simulink model "IMpanel"  (R2020a)
settings: Solver=ode45  StartTime=0.0  StopTime=10.0  FixedStep=5e-6  RelTol=1e-6  AbsTol=1e-8
values from neighbouring files (symbols this model uses):
  B = 0.08    [Mainprog.m]
  Ba = alphas * Jhat - Bhat    (= 0.17)    [Mainprog.m]
  Cdc = 5*470e-6    (= 0.00235)    [Mainprog.m]
  Flux_ref = 0.66*sqrt(2)*Lm/Lr    [Mainprog.m]
  Flux_ref_time = 0.001    [Mainprog.m]
  Israted = 9.1*sqrt(2)*1.2    [Mainprog.m]
  J = 0.05*0.25    (= 0.0125)    [Mainprog.m]
  kic = alphac * (RRhat + Rshat + Ra)    (= 15552.4475524)    [Mainprog.m]
  kis = alphas * (Bhat + Ba)    (= 5)    [Mainprog.m]
  kpc = alphac * Lsigmahat    (= 15.5524475524)    [Mainprog.m]
  kps = alphas * Jhat    (= 0.25)    [Mainprog.m]
  Lm = 0.135    [Mainprog.m]
  LMhat = LM    (= 0.127447552448)    [Mainprog.m]
  Lr = Lm+Lrl    (= 0.143)    [Mainprog.m]    (also in asymach.m = Lm+Lrl)
  Lrl = 0.008    [Mainprog.m]
  Lsigmahat = Lsigma    (= 0.0155524475524)    [Mainprog.m]
  Lsl = 0.008    [Mainprog.m]
  np = 2    [Mainprog.m]
  Ra = Lsigmahat * alphac - Rshat - RRhat    (= 13.1173079368)    [Mainprog.m]
  Rbatt = 1    [Mainprog.m]
  RR = (Lm/Lr)^2*Rr    (= 1.10513961563)    [Mainprog.m]
  Rr = 1.24    [Mainprog.m]
  RRhat = RR    (= 1.10513961563)    [Mainprog.m]
  Rs = 1.33    [Mainprog.m]
  speed_ref = 1435*pi/30    (= 150.272848597)    [Mainprog.m]
  speed_ref_time = 0.5    [Mainprog.m]
  Te_ref_time = 0.5    [Mainprog.m]
  Te_ref_value = 12    [Mainprog.m]
  TL_extra = 14.4    [Mainprog.m]    (also in asymach.m = u(3))
  TL_extra_time = 1    [Mainprog.m]
  Ts = 1/5000    (= 0.0002)    [Mainprog.m]
  Vbatt = 625    [Mainprog.m]
  Vdc0 = Vbatt    (= 625)    [Mainprog.m]
  xi = [0;0;0;0;0;0]    [Mainprog.m]
undefined symbols (not defined in the file or in its folder): j
libraries: simulink x1
settings Model: ExtModeTrigMode=oneshot  ExtModeArmWhenConnect=off  ExtModeAutoUpdateStatusClock=off  Creator=e6zebra  LastModifiedBy=miche
settings SolverCC: AutoScaleAbsTol=off
settings DataIOCC: SaveFormat=Array  SignalLoggingSaveFormat=ModelDataLogs  ReturnWorkspaceOutputs=off
settings OptimizationCC: BlockReduction=off  BooleanDataType=off  ExpressionDepthLimit=2147483647  InitFltsAndDblsToZero=on  LifeSpan=inf
settings DebuggingCC: SaveWithParameterizedLinksMsg=none  UnderspecifiedInitializationDetection=Classic  MergeDetectMultiDrivingBlocksExec=none  SignalResolutionControl=TryResolveAllWithWarning  MultiTaskDSMMsg=warning  MultiTaskCondExecSysMsg=none  FcnCallInpInsideContextMsg=warning  StateNameClashWarn=warning  SFUnexpectedBacktrackingDiag=warning  SFNoUnconditionalDefaultTransitionDiag=warning  SFExecutionAtInitializationDiag=none  ArithmeticOperatorsInVariantConditions=warning
settings HardwareCC: ProdBitPerPointer=32  ProdBitPerSizeT=32  ProdBitPerPtrDiffT=32  ProdLargestAtomicFloat=None  ProdIntDivRoundTo=Undefined  ProdEndianess=Unspecified  ProdWordSize=32  ProdHWDeviceType=32-bit Generic  TargetUnknown=on
settings ModelReferenceCC: PropagateSignalLabelsOutOfModel=off
settings SFSimCC: SimUseLocalCustomCode=off  CustomCodeUndefinedFunction=UseInterfaceOnly
settings RTWCC: TemplateMakefile=grt.tmf  RTWUseLocalCustomCode=off
settings CodeAppCC: StateflowObjectComments=on
settings GRTTargetCC: TargetFcnLib=ansi_tfl_tmw.mat  TargetLangStandard=C89/C90 (ANSI)  CombineOutputUpdateFcns=off  GRTInterface=on
settings ConfigComp: CovMetricSettings=dw  CovHtmlReporting=on  CovSaveCumulativeToWorkspaceVar=on  CovSaveSingleToWorkspaceVar=on  CovExternalEMLEnable=off  CovSFcnEnable=off

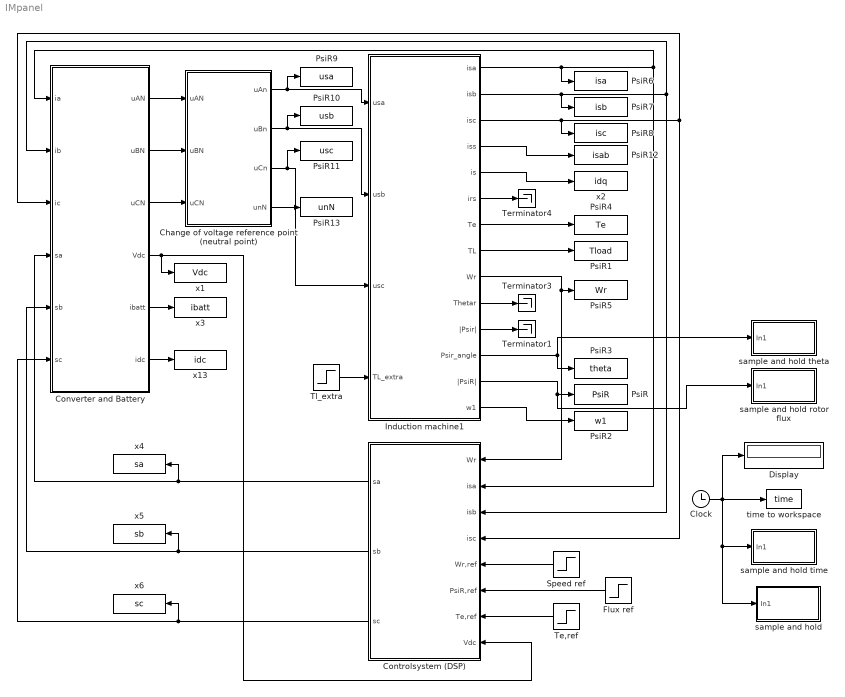
== system IMpanel ==
  Change of voltage reference point (neutral point) : Subsystem
  Clock : Clock
  Controlsystem (DSP) : Subsystem  TreatAsAtomicUnit=on
  Converter and Battery : Subsystem
  Display : Display
  Flux ref : Step  Time=Flux_ref_time  After=Flux_ref  SampleTime=0
  Induction machine1 : Subsystem
  PsiR : ToWorkspace  VariableName=PsiR  SampleTime=-1
  PsiR1 : ToWorkspace  VariableName=Tload  SampleTime=-1
  PsiR10 : ToWorkspace  VariableName=usb  SampleTime=-1
  PsiR11 : ToWorkspace  VariableName=usc  SampleTime=-1
  PsiR12 : ToWorkspace  VariableName=isab  SampleTime=-1
  PsiR13 : ToWorkspace  VariableName=unN  SampleTime=-1
  PsiR2 : ToWorkspace  VariableName=w1  SampleTime=-1
  PsiR3 : ToWorkspace  VariableName=theta  SampleTime=-1
  PsiR4 : ToWorkspace  VariableName=Te  SampleTime=-1
  PsiR5 : ToWorkspace  VariableName=Wr  SampleTime=-1
  PsiR6 : ToWorkspace  VariableName=isa  SampleTime=-1
  PsiR7 : ToWorkspace  VariableName=isb  SampleTime=-1
  PsiR8 : ToWorkspace  VariableName=isc  SampleTime=-1
  PsiR9 : ToWorkspace  VariableName=usa  SampleTime=-1
  Speed ref : Step  Time=speed_ref_time  After=speed_ref  SampleTime=0
  Te,ref : Step  Time=Te_ref_time  After=Te_ref_value  SampleTime=0
  Terminator1 : Terminator
  Terminator3 : Terminator
  Terminator4 : Terminator
  Tl_extra : Step  Time=TL_extra_time  After=TL_extra  SampleTime=0
  sample and hold : Subsystem
  sample and hold rotor flux : Subsystem
  sample and hold theta : Subsystem
  sample and hold time : Subsystem
  time to workspace : ToWorkspace  VariableName=time  SampleTime=-1
  x1 : ToWorkspace  VariableName=Vdc  SampleTime=-1
  x13 : ToWorkspace  VariableName=idc  SampleTime=-1
  x2 : ToWorkspace  VariableName=idq  SampleTime=-1
  x3 : ToWorkspace  VariableName=ibatt  SampleTime=-1
  x4 : ToWorkspace  VariableName=sa  SampleTime=-1
  x5 : ToWorkspace  VariableName=sb  SampleTime=-1
  x6 : ToWorkspace  VariableName=sc  SampleTime=-1
  wires:
  Clock/1 -> time to workspace/1, Display/1, sample and hold/1(In1), sample and hold time/1(In1)
  Induction machine1/13(|PsiR|) -> sample and hold rotor flux/1(In1), PsiR/1
  Induction machine1/9(Wr) -> Controlsystem (DSP)/1(Wr), PsiR5/1
  Induction machine1/3(isc) -> PsiR8/1, Controlsystem (DSP)/4(isc), Converter and Battery/3(ic)
  Induction machine1/2(isb) -> PsiR7/1, Controlsystem (DSP)/3(isb), Converter and Battery/2(ib)
  Induction machine1/1(isa) -> PsiR6/1, Controlsystem (DSP)/2(isa), Converter and Battery/1(ia)
  Flux ref/1 -> Controlsystem (DSP)/6(PsiR,ref)
  Speed ref/1 -> Controlsystem (DSP)/5(Wr,ref)
  Te,ref/1 -> Controlsystem (DSP)/7(Te,ref)
  Converter and Battery/5(ibatt) -> x3/1
  Converter and Battery/6(idc) -> x13/1
  Converter and Battery/4(Vdc) -> Controlsystem (DSP)/8(Vdc), x1/1
  Controlsystem (DSP)/1(sa) -> x4/1, Converter and Battery/4(sa)
  Controlsystem (DSP)/2(sb) -> x5/1, Converter and Battery/5(sb)
  Controlsystem (DSP)/3(sc) -> x6/1, Converter and Battery/6(sc)
  Converter and Battery/1(uAN) -> Change of voltage reference point (neutral point)/1(uAN)
  Converter and Battery/2(uBN) -> Change of voltage reference point (neutral point)/2(uBN)
  Converter and Battery/3(uCN) -> Change of voltage reference point (neutral point)/3(uCN)
  Change of voltage reference point (neutral point)/1(uAn) -> PsiR9/1, Induction machine1/1(usa)
  Change of voltage reference point (neutral point)/2(uBn) -> PsiR10/1, Induction machine1/2(usb)
  Change of voltage reference point (neutral point)/3(uCn) -> PsiR11/1, Induction machine1/3(usc)
  Change of voltage reference point (neutral point)/4(unN) -> PsiR13/1
  Induction machine1/7(Te) -> PsiR4/1
  Tl_extra/1 -> Induction machine1/4(TL_extra)
  Induction machine1/4(iss) -> PsiR12/1
  Induction machine1/5(is) -> x2/1
  Induction machine1/14(w1) -> PsiR2/1
  Induction machine1/8(TL) -> PsiR1/1
  Induction machine1/12(Psir_angle) -> sample and hold theta/1(In1), PsiR3/1
  Induction machine1/11(|Psir|) -> Terminator1/1
  Induction machine1/10(Thetar) -> Terminator3/1
  Induction machine1/6(irs) -> Terminator4/1

== system IMpanel/Change of voltage reference point (neutral point) ==
  uAN : Inport
  uBN : Inport  Port=2
  uCN : Inport  Port=3
  Gain2 : Gain  Gain=1/3  SaturateOnIntegerOverflow=on  OutDataTypeStr=Inherit: Same as input  ParamDataTypeStr=Inherit: Same as input
  Sum1 : Sum  Inputs=|+-  SaturateOnIntegerOverflow=on
  Sum4 : Sum  Inputs=|+-  SaturateOnIntegerOverflow=on
  Sum5 : Sum  Inputs=|+-  SaturateOnIntegerOverflow=on
  Sum7 : Sum  Inputs=+++  SaturateOnIntegerOverflow=on
  uAn : Outport  VectorParamsAs1DForOutWhenUnconnected=off
  uBn : Outport  Port=2  VectorParamsAs1DForOutWhenUnconnected=off
  uCn : Outport  Port=3  VectorParamsAs1DForOutWhenUnconnected=off
  unN : Outport  Port=4  VectorParamsAs1DForOutWhenUnconnected=off
  wires:
  uCN/1 -> Sum5/1, Sum7/1
  uBN/1 -> Sum4/1, Sum7/2
  uAN/1 -> Sum1/1, Sum7/3
  Sum7/1 -> Gain2/1
  Gain2/1 -> Sum1/2, Sum4/2, Sum5/2, unN/1
  Sum1/1 -> uAn/1
  Sum4/1 -> uBn/1
  Sum5/1 -> uCn/1

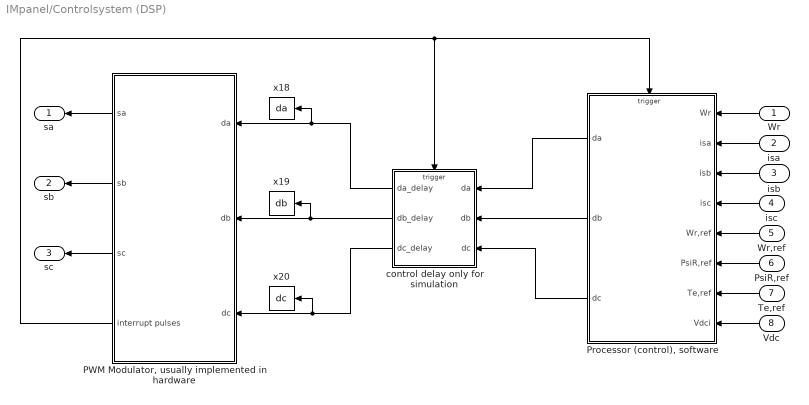
== system IMpanel/Controlsystem (DSP) ==
  Wr : Inport
  isa : Inport  Port=2
  isb : Inport  Port=3
  isc : Inport  Port=4
  Wr,ref : Inport  Port=5
  PsiR,ref : Inport  Port=6
  Te,ref : Inport  Port=7
  Vdc : Inport  Port=8
  "PWM Modulator, usually implemented in hardware" : Subsystem
  "Processor (control), software" : Subsystem  TreatAsAtomicUnit=on
  control delay only for simulation : Subsystem  TreatAsAtomicUnit=on
  x18 : ToWorkspace  VariableName=da  SampleTime=-1
  x19 : ToWorkspace  VariableName=db  SampleTime=-1
  x20 : ToWorkspace  VariableName=dc  SampleTime=-1
  sa : Outport  VectorParamsAs1DForOutWhenUnconnected=off
  sb : Outport  Port=2  VectorParamsAs1DForOutWhenUnconnected=off
  sc : Outport  Port=3  VectorParamsAs1DForOutWhenUnconnected=off
  wires:
  "PWM Modulator, usually implemented in hardware"/1(sa) -> sa/1
  "PWM Modulator, usually implemented in hardware"/2(sb) -> sb/1
  "PWM Modulator, usually implemented in hardware"/3(sc) -> sc/1
  Vdc/1 -> "Processor (control), software"/8(Vdci)
  Te,ref/1 -> "Processor (control), software"/7(Te,ref)
  PsiR,ref/1 -> "Processor (control), software"/6(PsiR,ref)
  Wr,ref/1 -> "Processor (control), software"/5(Wr,ref)
  Wr/1 -> "Processor (control), software"/1(Wr)
  isa/1 -> "Processor (control), software"/2(isa)
  isb/1 -> "Processor (control), software"/3(isb)
  isc/1 -> "Processor (control), software"/4(isc)
  "PWM Modulator, usually implemented in hardware"/4("interrupt pulses ") -> "Processor (control), software"/Trigger, control delay only for simulation/Trigger
  "Processor (control), software"/1(da) -> control delay only for simulation/1(da)
  control delay only for simulation/1(da_delay) -> x18/1, "PWM Modulator, usually implemented in hardware"/1(da)
  "Processor (control), software"/2(db) -> control delay only for simulation/2(db)
  control delay only for simulation/2(db_delay) -> x19/1, "PWM Modulator, usually implemented in hardware"/2(db)
  "Processor (control), software"/3(dc) -> control delay only for simulation/3(dc)
  control delay only for simulation/3(dc_delay) -> x20/1, "PWM Modulator, usually implemented in hardware"/3(dc)

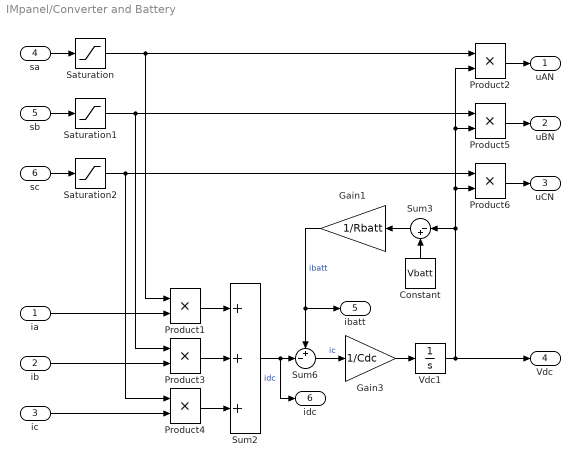
== system IMpanel/Converter and Battery ==
  ia : Inport
  ib : Inport  Port=2
  ic : Inport  Port=3
  sa : Inport  Port=4
  sb : Inport  Port=5
  sc : Inport  Port=6
  Constant : Constant  Value=Vbatt
  Gain1 : Gain  Gain=1/Rbatt  SaturateOnIntegerOverflow=on  OutDataTypeStr=Inherit: Same as input  ParamDataTypeStr=Inherit: Same as input
  Gain3 : Gain  Gain=1/Cdc  SaturateOnIntegerOverflow=on  OutDataTypeStr=Inherit: Same as input  ParamDataTypeStr=Inherit: Same as input
  Product{1..6} (6 alike) : Product  SaturateOnIntegerOverflow=on  OutDataTypeStr=Inherit: Same as first input
  Saturation : Saturate  UpperLimit=1.0  LowerLimit=0.0
  Saturation1 : Saturate  UpperLimit=1.0  LowerLimit=0.0
  Saturation2 : Saturate  UpperLimit=1.0  LowerLimit=0.0
  Sum2 : Sum  Inputs=+++  SaturateOnIntegerOverflow=on
  Sum3 : Sum  Inputs=|-+  SaturateOnIntegerOverflow=on
  Sum6 : Sum  Inputs=+-|  SaturateOnIntegerOverflow=on
  Vdc1 : Integrator  InitialCondition=Vdc0  LimitOutput=on  LowerSaturationLimit=1
  uAN : Outport  VectorParamsAs1DForOutWhenUnconnected=off
  uBN : Outport  Port=2  VectorParamsAs1DForOutWhenUnconnected=off
  uCN : Outport  Port=3  VectorParamsAs1DForOutWhenUnconnected=off
  Vdc : Outport  Port=4  VectorParamsAs1DForOutWhenUnconnected=off
  ibatt : Outport  Port=5  VectorParamsAs1DForOutWhenUnconnected=off
  idc : Outport  Port=6  VectorParamsAs1DForOutWhenUnconnected=off
  wires:
  Product2/1 -> uAN/1
  ic/1 -> Product4/2
  ib/1 -> Product3/2
  ia/1 -> Product1/2
  sa/1 -> Saturation/1
  sb/1 -> Saturation1/1
  sc/1 -> Saturation2/1
  Saturation2/1 -> Product4/1, Product6/1
  Saturation1/1 -> Product3/1, Product5/1
  Saturation/1 -> Product1/1, Product2/1
  Vdc1/1 -> Vdc/1, Sum3/1, Product6/2, Product5/2, Product2/2
  Constant/1 -> Sum3/2
  Product5/1 -> uBN/1
  Product6/1 -> uCN/1
  Product1/1 -> Sum2/1
  Product3/1 -> Sum2/2
  Product4/1 -> Sum2/3
  Sum3/1 -> Gain1/1
  Sum6/1 -> Gain3/1  "ic"
  Sum2/1 -> Sum6/2, idc/1  "idc"
  Gain1/1 -> Sum6/1, ibatt/1  "ibatt"
  Gain3/1 -> Vdc1/1

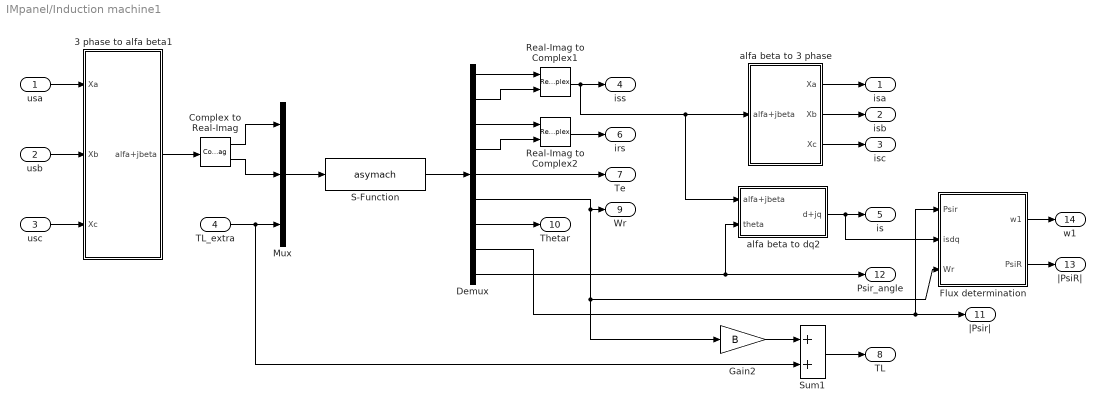
== system IMpanel/Induction machine1 ==
  usa : Inport
  usb : Inport  Port=2
  usc : Inport  Port=3
  TL_extra : Inport  Port=4
  3 phase to alfa beta1 : Subsystem
  Complex to Real-Imag : ComplexToRealImag
  Demux : Demux  Outputs=9
      settings: DisplayOption=none
  Flux determination : Subsystem
  Gain2 : Gain  Gain=B
  Mux : Mux  Inputs=3
  Real-Imag to Complex1 : RealImagToComplex
  Real-Imag to Complex2 : RealImagToComplex
  S-Function : S-Function  FunctionName=asymach  Parameters=Rs,Rr,Lm,Lsl,Lrl,J,np,B,xi  SFunctionDeploymentMode=off  EnableBusSupport=off
  Sum1 : Sum  InputSameDT=on  SaturateOnIntegerOverflow=on  OutDataTypeStr=Inherit: Same as first input
  alfa beta to 3 phase : Subsystem
  alfa beta to dq2 : Subsystem
  isa : Outport  VectorParamsAs1DForOutWhenUnconnected=off
  isb : Outport  Port=2  VectorParamsAs1DForOutWhenUnconnected=off
  isc : Outport  Port=3  VectorParamsAs1DForOutWhenUnconnected=off
  iss : Outport  Port=4  VectorParamsAs1DForOutWhenUnconnected=off
  is : Outport  Port=5  VectorParamsAs1DForOutWhenUnconnected=off
  irs : Outport  Port=6  VectorParamsAs1DForOutWhenUnconnected=off
  Te : Outport  Port=7  VectorParamsAs1DForOutWhenUnconnected=off
  TL : Outport  Port=8  VectorParamsAs1DForOutWhenUnconnected=off
  Wr : Outport  Port=9  VectorParamsAs1DForOutWhenUnconnected=off
  Thetar : Outport  Port=10  VectorParamsAs1DForOutWhenUnconnected=off
  |Psir| : Outport  Port=11  VectorParamsAs1DForOutWhenUnconnected=off
  Psir_angle : Outport  Port=12  VectorParamsAs1DForOutWhenUnconnected=off
  |PsiR| : Outport  Port=13  VectorParamsAs1DForOutWhenUnconnected=off
  w1 : Outport  Port=14  VectorParamsAs1DForOutWhenUnconnected=off
  wires:
  TL_extra/1 -> Mux/3, Sum1/2
  S-Function/1 -> Demux/1
  Mux/1 -> S-Function/1
  Demux/1 -> Real-Imag to Complex1/1
  Demux/2 -> Real-Imag to Complex1/2
  Real-Imag to Complex1/1 -> iss/1, alfa beta to dq2/1(alfa+jbeta), alfa beta to 3 phase/1(alfa+jbeta)
  Demux/3 -> Real-Imag to Complex2/1
  Demux/4 -> Real-Imag to Complex2/2
  Complex to Real-Imag/2 -> Mux/2
  Complex to Real-Imag/1 -> Mux/1
  alfa beta to dq2/1(d+jq) -> is/1, Flux determination/2(isdq)
  Real-Imag to Complex2/1 -> irs/1
  Demux/5 -> Te/1
  Sum1/1 -> TL/1
  Gain2/1 -> Sum1/1
  Demux/6 -> Wr/1, Gain2/1, Flux determination/3(Wr)
  Demux/7 -> Thetar/1
  Demux/9 -> alfa beta to dq2/2(theta), Psir_angle/1
  Demux/8 -> |Psir|/1, Flux determination/1(Psir)
  3 phase to alfa beta1/1(alfa+jbeta) -> Complex to Real-Imag/1
  usc/1 -> 3 phase to alfa beta1/3(Xc)
  usb/1 -> 3 phase to alfa beta1/2(Xb)
  usa/1 -> 3 phase to alfa beta1/1(Xa)
  alfa beta to 3 phase/1(Xa) -> isa/1
  alfa beta to 3 phase/3(Xc) -> isc/1
  alfa beta to 3 phase/2(Xb) -> isb/1
  Flux determination/2(PsiR) -> |PsiR|/1
  Flux determination/1(w1) -> w1/1

== system IMpanel/sample and hold ==
  In1 : Inport
  Pulse Generator : DiscretePulseGenerator  PulseType=Time based  Period=Ts/2  PulseWidth=50
  control : Subsystem  TreatAsAtomicUnit=on
  wires:
  Pulse Generator/1 -> control/Trigger
  In1/1 -> control/1(in)

== system IMpanel/sample and hold rotor flux ==
  In1 : Inport
  Pulse Generator : DiscretePulseGenerator  PulseType=Time based  Period=Ts  PulseWidth=50
  control : Subsystem  TreatAsAtomicUnit=on
  wires:
  In1/1 -> control/1(in)
  Pulse Generator/1 -> control/Trigger

== system IMpanel/sample and hold theta ==
  In1 : Inport
  Pulse Generator : DiscretePulseGenerator  PulseType=Time based  Period=Ts  PulseWidth=50
  control : Subsystem  TreatAsAtomicUnit=on
  wires:
  Pulse Generator/1 -> control/Trigger
  In1/1 -> control/1(in)

== system IMpanel/sample and hold time ==
  In1 : Inport
  Pulse Generator : DiscretePulseGenerator  PulseType=Time based  Period=Ts  PulseWidth=50
  control : Subsystem  TreatAsAtomicUnit=on
  wires:
  Pulse Generator/1 -> control/Trigger
  In1/1 -> control/1(in)

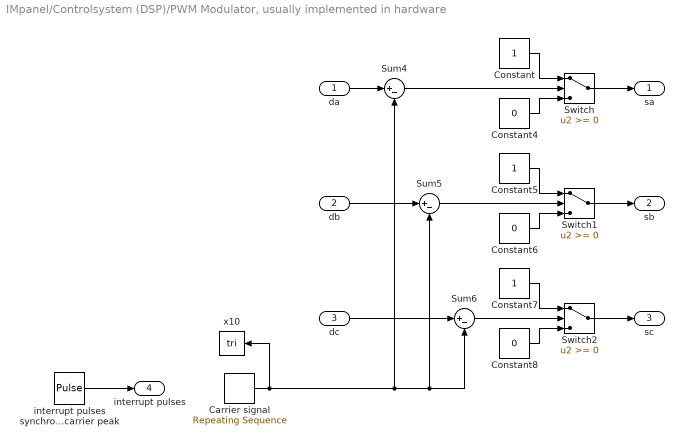
== system IMpanel/Controlsystem (DSP)/PWM Modulator, usually implemented in hardware ==
  da : Inport
  db : Inport  Port=2
  dc : Inport  Port=3
  Carrier signal : simulink/Sources/Repeating Sequence  rep_seq_t=[0 Ts/2 Ts]  rep_seq_y=[0 1 0]
  Constant : Constant
  Constant4 : Constant  Value=0
  Constant5 : Constant
  Constant6 : Constant  Value=0
  Constant7 : Constant
  Constant8 : Constant  Value=0
  Sum4 : Sum  Inputs=|+-
  Sum5 : Sum  Inputs=|+-
  Sum6 : Sum  Inputs=|+-
  Switch : Switch
  Switch1 : Switch
  Switch2 : Switch
  interrupt pulses synchronized with the carrier peak : DiscretePulseGenerator  PulseType=Time based  Period=Ts  PulseWidth=50
  x10 : ToWorkspace  VariableName=tri  SampleTime=-1
  sa : Outport  VectorParamsAs1DForOutWhenUnconnected=off
  sb : Outport  Port=2  VectorParamsAs1DForOutWhenUnconnected=off
  sc : Outport  Port=3  VectorParamsAs1DForOutWhenUnconnected=off
  "interrupt pulses " : Outport  Port=4  VectorParamsAs1DForOutWhenUnconnected=off
  wires:
  Constant/1 -> Switch/1
  Constant4/1 -> Switch/3
  Sum4/1 -> Switch/2
  Constant5/1 -> Switch1/1
  Constant6/1 -> Switch1/3
  Sum5/1 -> Switch1/2
  Constant7/1 -> Switch2/1
  Constant8/1 -> Switch2/3
  Sum6/1 -> Switch2/2
  Carrier signal/1 -> Sum6/2, Sum5/2, Sum4/2, x10/1
  Switch/1 -> sa/1
  Switch2/1 -> sc/1
  Switch1/1 -> sb/1
  da/1 -> Sum4/1
  db/1 -> Sum5/1
  dc/1 -> Sum6/1
  interrupt pulses synchronized with the carrier peak/1 -> "interrupt pulses "/1

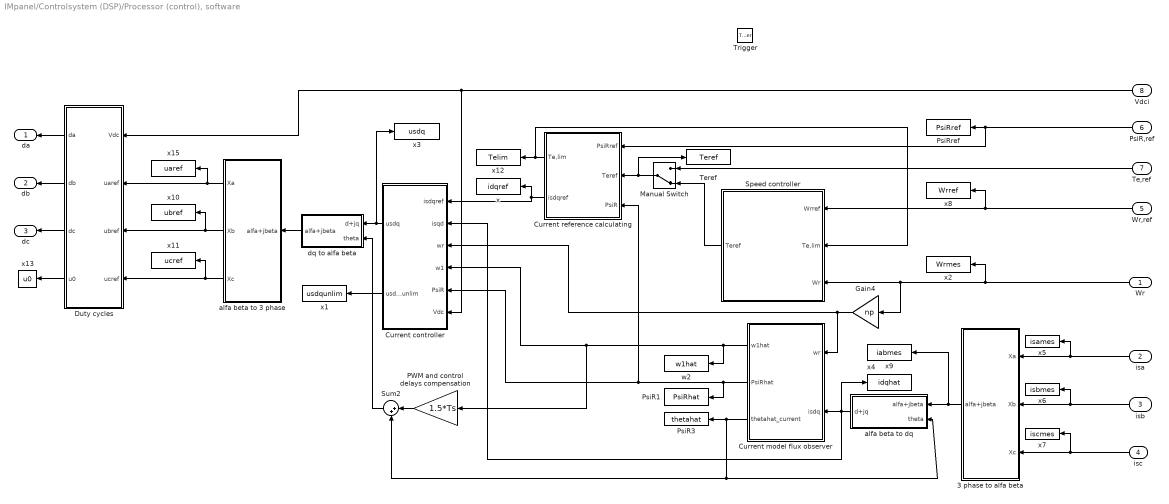
== system IMpanel/Controlsystem (DSP)/Processor (control), software ==
  Wr : Inport
  isa : Inport  Port=2
  isb : Inport  Port=3
  isc : Inport  Port=4
  Wr,ref : Inport  Port=5
  PsiR,ref : Inport  Port=6
  Te,ref : Inport  Port=7
  Vdci : Inport  Port=8
  Trigger : TriggerPort  VariantControl=(inherit)
  " Current model flux observer" : Subsystem
  3 phase to alfa beta : Subsystem
  Current controller : Subsystem
  Current reference calculating : Subsystem
  Duty cycles : Subsystem
  Gain4 : Gain  Gain=np  SaturateOnIntegerOverflow=on  OutDataTypeStr=Inherit: Same as input  ParamDataTypeStr=Inherit: Same as input
  Manual Switch : ManualSwitch  CurrentSetting=0
  PWM and control delays compensation : Gain  Gain=1.5*Ts  SaturateOnIntegerOverflow=on  OutDataTypeStr=Inherit: Same as input  ParamDataTypeStr=Inherit: Same as input
  PsiR1 : ToWorkspace  VariableName=PsiRhat  SampleTime=-1
  PsiR3 : ToWorkspace  VariableName=thetahat  SampleTime=-1
  PsiRref : ToWorkspace  VariableName=PsiRref  SampleTime=-1
  Speed controller : Subsystem
  Sum2 : Sum  Inputs=|++  SaturateOnIntegerOverflow=on
  Teref : ToWorkspace  VariableName=Teref  SampleTime=-1
  alfa beta to 3 phase : Subsystem
  alfa beta to dq : Subsystem
  dq to alfa beta : Subsystem
  w2 : ToWorkspace  VariableName=w1hat  SampleTime=-1
  x : ToWorkspace  VariableName=idqref  SampleTime=-1
  x1 : ToWorkspace  VariableName=usdqunlim  SampleTime=-1
  x10 : ToWorkspace  VariableName=ubref  SampleTime=-1
  x11 : ToWorkspace  VariableName=ucref  SampleTime=-1
  x12 : ToWorkspace  VariableName=Telim  SampleTime=-1
  x13 : ToWorkspace  VariableName=u0  SampleTime=-1
  x15 : ToWorkspace  VariableName=uaref  SampleTime=-1
  x2 : ToWorkspace  VariableName=Wrmes  SampleTime=-1
  x3 : ToWorkspace  VariableName=usdq  SampleTime=-1
  x4 : ToWorkspace  VariableName=idqhat  SampleTime=-1
  x5 : ToWorkspace  VariableName=isames  SampleTime=-1
  x6 : ToWorkspace  VariableName=isbmes  SampleTime=-1
  x7 : ToWorkspace  VariableName=iscmes  SampleTime=-1
  x8 : ToWorkspace  VariableName=Wrref  SampleTime=-1
  x9 : ToWorkspace  VariableName=iabmes  SampleTime=-1
  da : Outport  VectorParamsAs1DForOutWhenUnconnected=off
  db : Outport  Port=2  VectorParamsAs1DForOutWhenUnconnected=off
  dc : Outport  Port=3  VectorParamsAs1DForOutWhenUnconnected=off
  wires:
  Current controller/1(usdq) -> x3/1, dq to alfa beta/1(d+jq)
  " Current model flux observer"/2(PsiRhat) -> Current controller/5(PsiR), Current reference calculating/3(PsiR), PsiR1/1
  " Current model flux observer"/1(w1hat) -> w2/1, Current controller/4(w1), PWM and control delays compensation/1
  dq to alfa beta/1(alfa+jbeta) -> alfa beta to 3 phase/1(alfa+jbeta)
  Current controller/2(usdq unlim) -> x1/1
  alfa beta to dq/1(d+jq) -> " Current model flux observer"/2(isdq), x4/1, Current controller/2(isqd)
  Current reference calculating/1(Te,lim) -> Speed controller/2(Te,lim), x12/1
  Wr,ref/1 -> Speed controller/1(Wrref), x8/1
  3 phase to alfa beta/1(alfa+jbeta) -> alfa beta to dq/1(alfa+jbeta), x9/1
  Wr/1 -> x2/1, Speed controller/3(Wr), Gain4/1
  " Current model flux observer"/3(thetahat_current) -> PsiR3/1, Sum2/2, alfa beta to dq/2(theta)
  alfa beta to 3 phase/3(Xc) -> x11/1, Duty cycles/4(ucref)
  alfa beta to 3 phase/2(Xb) -> Duty cycles/3(ubref), x10/1
  alfa beta to 3 phase/1(Xa) -> x15/1, Duty cycles/2(uaref)
  Vdci/1 -> Duty cycles/1(Vdc), Current controller/6(Vdc)
  Gain4/1 -> Current controller/3(wr), " Current model flux observer"/1(wr)
  Manual Switch/1 -> Current reference calculating/2(Teref), Teref/1
  Speed controller/1(Teref) -> Manual Switch/2
  Te,ref/1 -> Manual Switch/1
  isa/1 -> 3 phase to alfa beta/1(Xa), x5/1
  isb/1 -> 3 phase to alfa beta/2(Xb), x6/1
  isc/1 -> 3 phase to alfa beta/3(Xc), x7/1
  PsiR,ref/1 -> PsiRref/1, Current reference calculating/1(PsiRref)
  Current reference calculating/2(isdqref) -> Current controller/1(isdqref), x/1
  Sum2/1 -> dq to alfa beta/2(theta)
  PWM and control delays compensation/1 -> Sum2/1
  Duty cycles/1(da) -> da/1
  Duty cycles/2(db) -> db/1
  Duty cycles/3(dc) -> dc/1
  Duty cycles/4(u0) -> x13/1

== system IMpanel/Controlsystem (DSP)/control delay only for simulation ==
  da : Inport
  db : Inport  Port=2
  dc : Inport  Port=3
  Trigger : TriggerPort  VariantControl=(inherit)
  Unit Delay : UnitDelay  InitialCondition=0.5  SampleTime=-1  HasFrameUpgradeWarning=on
  Unit Delay1 : UnitDelay  InitialCondition=0.5  SampleTime=-1  HasFrameUpgradeWarning=on
  Unit Delay2 : UnitDelay  InitialCondition=0.5  SampleTime=-1  HasFrameUpgradeWarning=on
  da_delay : Outport  InitialOutput=[0]  VectorParamsAs1DForOutWhenUnconnected=off
  db_delay : Outport  Port=2  InitialOutput=[0]  VectorParamsAs1DForOutWhenUnconnected=off
  dc_delay : Outport  Port=3  InitialOutput=[0]  VectorParamsAs1DForOutWhenUnconnected=off
  wires:
  da/1 -> Unit Delay/1
  Unit Delay/1 -> da_delay/1
  Unit Delay1/1 -> db_delay/1
  db/1 -> Unit Delay1/1
  dc/1 -> Unit Delay2/1
  Unit Delay2/1 -> dc_delay/1

== system IMpanel/Induction machine1/3 phase to alfa beta1 ==
  Xa : Inport
  Xb : Inport  Port=2
  Xc : Inport  Port=3
  Add : Sum  Inputs=+--
  Add1 : Sum  Inputs=+-
  Add2 : Sum
  Gain : Gain  Gain=j/sqrt(3)
  Gain1 : Gain  Gain=2/3
  Gain2 : Gain  Gain=1/3
  Gain3 : Gain  Gain=1/3
  alfa+jbeta : Outport  VectorParamsAs1DForOutWhenUnconnected=off
  wires:
  Add1/1 -> Gain/1
  Add2/1 -> alfa+jbeta/1
  Gain/1 -> Add2/2  "beta"
  Add/1 -> Add2/1  "alfa"
  Gain3/1 -> Add/3
  Gain2/1 -> Add/2
  Gain1/1 -> Add/1
  Xa/1 -> Gain1/1
  Xb/1 -> Gain2/1, Add1/1
  Xc/1 -> Gain3/1, Add1/2

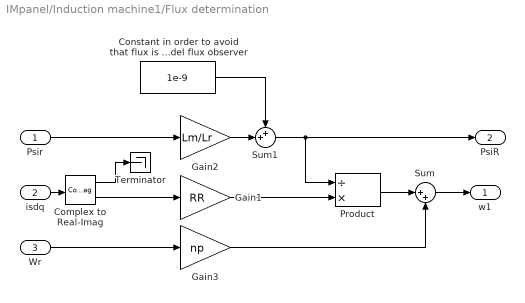
== system IMpanel/Induction machine1/Flux determination ==
  Psir : Inport
  isdq : Inport  Port=2
  Wr : Inport  Port=3
  Complex to Real-Imag : ComplexToRealImag
  "Constant in order to avoid that flux is equal to zero when dividing with it, for example in the current reference calculating block and in the current model flux observer" : Constant  Value=1e-9
  Gain1 : Gain  Gain=RR  SaturateOnIntegerOverflow=on  OutDataTypeStr=Inherit: Same as input  ParamDataTypeStr=Inherit: Same as input
  Gain2 : Gain  Gain=Lm/Lr  SaturateOnIntegerOverflow=on  OutDataTypeStr=Inherit: Same as input  ParamDataTypeStr=Inherit: Same as input
  Gain3 : Gain  Gain=np  SaturateOnIntegerOverflow=on  OutDataTypeStr=Inherit: Same as input  ParamDataTypeStr=Inherit: Same as input
  Product : Product  Inputs=/*  SaturateOnIntegerOverflow=on  OutDataTypeStr=Inherit: Same as first input
  Sum : Sum  Inputs=|++  SaturateOnIntegerOverflow=on
  Sum1 : Sum  Inputs=++|  SaturateOnIntegerOverflow=on
  Terminator : Terminator
  w1 : Outport  VectorParamsAs1DForOutWhenUnconnected=off
  PsiR : Outport  Port=2  VectorParamsAs1DForOutWhenUnconnected=off
  wires:
  Gain1/1 -> Product/2
  Product/1 -> Sum/1
  Sum/1 -> w1/1
  Wr/1 -> Gain3/1
  Psir/1 -> Gain2/1
  Sum1/1 -> PsiR/1, Product/1
  Gain3/1 -> Sum/2
  Complex to Real-Imag/1 -> Terminator/1
  isdq/1 -> Complex to Real-Imag/1
  Complex to Real-Imag/2 -> Gain1/1
  Gain2/1 -> Sum1/2
  "Constant in order to avoid that flux is equal to zero when dividing with it, for example in the current reference calculating block and in the current model flux observer"/1 -> Sum1/1

== system IMpanel/Induction machine1/alfa beta to 3 phase ==
  alfa+jbeta : Inport
  Add1 : Sum  Inputs=-+
  Add2 : Sum  Inputs=--
  Complex to Real-Imag : ComplexToRealImag
  Gain1 : Gain  Gain=sqrt(3)/2
  Gain2 : Gain  Gain=1/2
  Xa : Outport  VectorParamsAs1DForOutWhenUnconnected=off
  Xb : Outport  Port=2  VectorParamsAs1DForOutWhenUnconnected=off
  Xc : Outport  Port=3  VectorParamsAs1DForOutWhenUnconnected=off
  wires:
  alfa+jbeta/1 -> Complex to Real-Imag/1
  Complex to Real-Imag/1 -> Xa/1, Gain2/1
  Add2/1 -> Xc/1
  Add1/1 -> Xb/1
  Complex to Real-Imag/2 -> Gain1/1
  Gain1/1 -> Add1/2, Add2/2
  Gain2/1 -> Add1/1, Add2/1

== system IMpanel/Induction machine1/alfa beta to dq2 ==
  alfa+jbeta : Inport
  theta : Inport  Port=2
  Gain : Gain  Gain=-j  SaturateOnIntegerOverflow=on  OutDataTypeStr=Inherit: Same as input  ParamDataTypeStr=Inherit: Same as input
  Math Function : Math  SignedPower=on  SaturateOnIntegerOverflow=on
  Product : Product  SaturateOnIntegerOverflow=on  OutDataTypeStr=Inherit: Same as first input
  d+jq : Outport  VectorParamsAs1DForOutWhenUnconnected=off
  wires:
  theta/1 -> Gain/1
  Gain/1 -> Math Function/1
  Math Function/1 -> Product/2
  alfa+jbeta/1 -> Product/1
  Product/1 -> d+jq/1

== system IMpanel/sample and hold/control ==
  in : Inport
  Trigger : TriggerPort  VariantControl=(inherit)
  Terminator : Terminator
  wires:
  in/1 -> Terminator/1

== system IMpanel/sample and hold rotor flux/control ==
  in : Inport
  Trigger : TriggerPort  VariantControl=(inherit)
  time to workspace2 : ToWorkspace  VariableName=PsiR_dis  SampleTime=-1
  wires:
  in/1 -> time to workspace2/1

== system IMpanel/sample and hold theta/control ==
  in : Inport
  Trigger : TriggerPort  VariantControl=(inherit)
  time to workspace3 : ToWorkspace  VariableName=theta_dis  SampleTime=-1
  wires:
  in/1 -> time to workspace3/1

== system IMpanel/sample and hold time/control ==
  in : Inport
  Trigger : TriggerPort  VariantControl=(inherit)
  disc time to workspace : ToWorkspace  VariableName=time_dis  SampleTime=-1
  wires:
  in/1 -> disc time to workspace/1

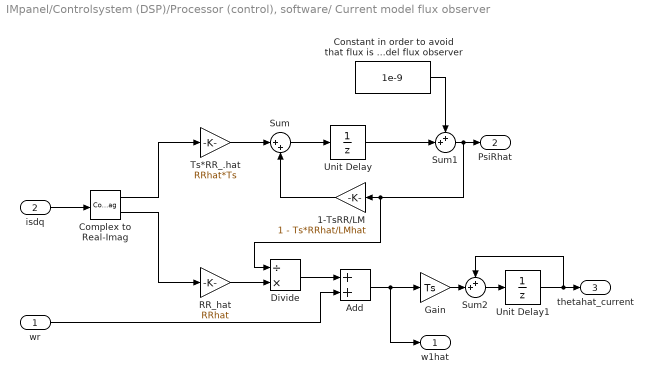
== system IMpanel/Controlsystem (DSP)/Processor (control), software/ Current model flux observer ==
  wr : Inport
  isdq : Inport  Port=2
  1-TsRR/LM : Gain  Gain=1 - Ts*RRhat/LMhat
  Add : Sum
  Complex to Real-Imag : ComplexToRealImag
  "Constant in order to avoid that flux is equal to zero when dividing with it, for example in the current reference calculating block and in the current model flux observer" : Constant  Value=1e-9  SampleTime=-1
  Divide : Product  Inputs=/*
  Gain : Gain  Gain=Ts
  RR_hat : Gain  Gain=RRhat
  Sum : Sum  Inputs=|++
  Sum1 : Sum  Inputs=++|  SaturateOnIntegerOverflow=on
  Sum2 : Sum  Inputs=++|
  Ts*RR_.hat : Gain  Gain=RRhat*Ts
  Unit Delay : UnitDelay  SampleTime=-1  HasFrameUpgradeWarning=on
  Unit Delay1 : UnitDelay  SampleTime=-1  HasFrameUpgradeWarning=on
  w1hat : Outport  VectorParamsAs1DForOutWhenUnconnected=off
  PsiRhat : Outport  Port=2  VectorParamsAs1DForOutWhenUnconnected=off
  thetahat_current : Outport  Port=3  VectorParamsAs1DForOutWhenUnconnected=off
  wires:
  "Constant in order to avoid that flux is equal to zero when dividing with it, for example in the current reference calculating block and in the current model flux observer"/1 -> Sum1/1
  Sum1/1 -> Divide/1, 1-TsRR/LM/1, PsiRhat/1
  Ts*RR_.hat/1 -> Sum/1
  Sum/1 -> Unit Delay/1
  Unit Delay/1 -> Sum1/2
  isdq/1 -> Complex to Real-Imag/1
  1-TsRR/LM/1 -> Sum/2
  Add/1 -> w1hat/1, Gain/1
  RR_hat/1 -> Divide/2
  Divide/1 -> Add/1
  Complex to Real-Imag/2 -> RR_hat/1
  wr/1 -> Add/2
  Complex to Real-Imag/1 -> Ts*RR_.hat/1
  Gain/1 -> Sum2/2
  Sum2/1 -> Unit Delay1/1
  Unit Delay1/1 -> thetahat_current/1, Sum2/1

== system IMpanel/Controlsystem (DSP)/Processor (control), software/3 phase to alfa beta ==
  Xa : Inport
  Xb : Inport  Port=2
  Xc : Inport  Port=3
  Add : Sum  Inputs=+--
  Add1 : Sum  Inputs=+-
  Add2 : Sum
  Gain : Gain  Gain=j/sqrt(3)
  Gain1 : Gain  Gain=2/3
  Gain2 : Gain  Gain=1/3
  Gain3 : Gain  Gain=1/3
  alfa+jbeta : Outport  VectorParamsAs1DForOutWhenUnconnected=off
  wires:
  Add1/1 -> Gain/1
  Add2/1 -> alfa+jbeta/1
  Gain/1 -> Add2/2  "beta"
  Add/1 -> Add2/1  "alfa"
  Gain3/1 -> Add/3
  Gain2/1 -> Add/2
  Gain1/1 -> Add/1
  Xa/1 -> Gain1/1
  Xb/1 -> Gain2/1, Add1/1
  Xc/1 -> Gain3/1, Add1/2

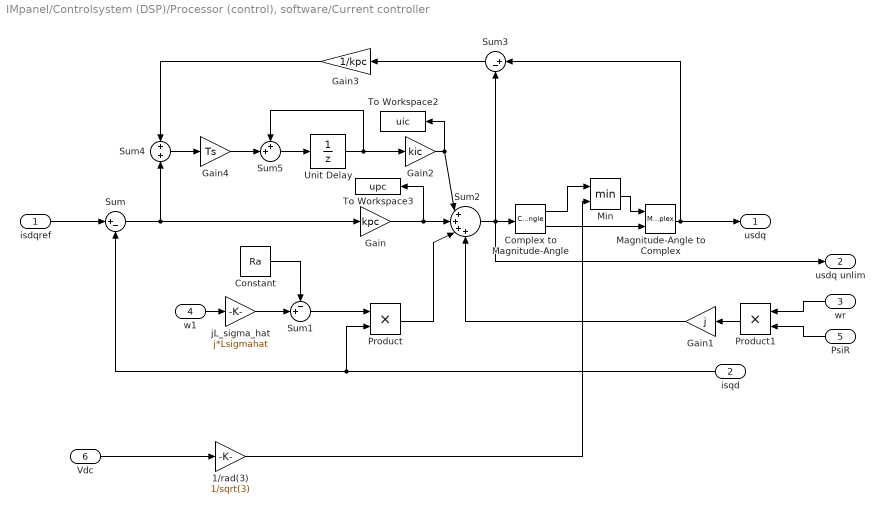
== system IMpanel/Controlsystem (DSP)/Processor (control), software/Current controller ==
  isdqref : Inport
  isqd : Inport  Port=2
  wr : Inport  Port=3
  w1 : Inport  Port=4
  PsiR : Inport  Port=5
  Vdc : Inport  Port=6
  1/rad(3) : Gain  Gain=1/sqrt(3)
  Complex to Magnitude-Angle : ComplexToMagnitudeAngle
  Constant : Constant  Value=Ra
  Gain : Gain  Gain=kpc
  Gain1 : Gain  Gain=j
  Gain2 : Gain  Gain=kic
  Gain3 : Gain  Gain=1/kpc
  Gain4 : Gain  Gain=Ts
  Magnitude-Angle to Complex : MagnitudeAngleToComplex
  Min : MinMax  Inputs=2
  Product : Product
  Product1 : Product
  Sum : Sum  Inputs=|+-
  Sum1 : Sum  Inputs=-+|
  Sum2 : Sum  Inputs=|++++
  Sum3 : Sum  Inputs=|+-
  Sum4 : Sum
  Sum5 : Sum  Inputs=++|
  To Workspace2 : ToWorkspace  VariableName=uic  SampleTime=-1
  To Workspace3 : ToWorkspace  VariableName=upc  SampleTime=-1
  Unit Delay : UnitDelay  SampleTime=-1  HasFrameUpgradeWarning=on
  jL_sigma_hat : Gain  Gain=j*Lsigmahat
  usdq : Outport  VectorParamsAs1DForOutWhenUnconnected=off
  usdq unlim : Outport  Port=2  VectorParamsAs1DForOutWhenUnconnected=off
  wires:
  Sum5/1 -> Unit Delay/1
  Sum/1 -> Gain/1, Sum4/2
  Magnitude-Angle to Complex/1 -> Sum3/1, usdq/1
  Gain/1 -> To Workspace3/1, Sum2/2
  Sum3/1 -> Gain3/1
  Sum2/1 -> Complex to Magnitude-Angle/1, usdq unlim/1, Sum3/2
  Gain3/1 -> Sum4/1
  Min/1 -> Magnitude-Angle to Complex/1
  Gain2/1 -> To Workspace2/1, Sum2/1
  Complex to Magnitude-Angle/1 -> Min/1
  Complex to Magnitude-Angle/2 -> Magnitude-Angle to Complex/2
  Gain4/1 -> Sum5/2
  Sum4/1 -> Gain4/1
  Unit Delay/1 -> Gain2/1, Sum5/1
  isdqref/1 -> Sum/1
  isqd/1 -> Sum/2, Product/2
  Product1/1 -> Gain1/1
  Product/1 -> Sum2/3
  Gain1/1 -> Sum2/4
  Sum1/1 -> Product/1
  wr/1 -> Product1/1
  Constant/1 -> Sum1/1
  PsiR/1 -> Product1/2
  jL_sigma_hat/1 -> Sum1/2
  w1/1 -> jL_sigma_hat/1
  Vdc/1 -> 1/rad(3)/1
  1/rad(3)/1 -> Min/2

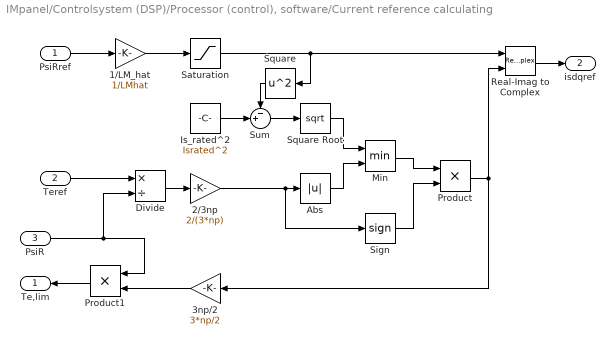
== system IMpanel/Controlsystem (DSP)/Processor (control), software/Current reference calculating ==
  PsiRref : Inport
  Teref : Inport  Port=2
  PsiR : Inport  Port=3
  1/LM_hat : Gain  Gain=1/LMhat
  2/3np : Gain  Gain=2/(3*np)
  3np/2 : Gain  Gain=3*np/2
  Abs : Abs
  Divide : Product  Inputs=*/
  Is_rated^2 : Constant  Value=Israted^2  SampleTime=-1
  Min : MinMax  Inputs=2
  Product : Product
  Product1 : Product
  Real-Imag to Complex : RealImagToComplex
  Saturation : Saturate  UpperLimit=Israted  LowerLimit=0
  Sign : Signum
  Square : Math  Operator=square  SaturateOnIntegerOverflow=on
  Square Root : Sqrt  SaturateOnIntegerOverflow=on
  Sum : Sum  Inputs=-+|
  Te,lim : Outport  VectorParamsAs1DForOutWhenUnconnected=off
  isdqref : Outport  Port=2  VectorParamsAs1DForOutWhenUnconnected=off
  wires:
  PsiRref/1 -> 1/LM_hat/1
  Real-Imag to Complex/1 -> isdqref/1
  Saturation/1 -> Square/1, Real-Imag to Complex/1
  Abs/1 -> Min/2
  Product1/1 -> Te,lim/1
  Teref/1 -> Divide/1
  Product/1 -> 3np/2/1, Real-Imag to Complex/2
  Sign/1 -> Product/2
  2/3np/1 -> Sign/1, Abs/1
  Min/1 -> Product/1
  Divide/1 -> 2/3np/1
  Is_rated^2/1 -> Sum/2
  3np/2/1 -> Product1/2
  Square/1 -> Sum/1
  1/LM_hat/1 -> Saturation/1
  PsiR/1 -> Divide/2, Product1/1
  Square Root/1 -> Min/1
  Sum/1 -> Square Root/1

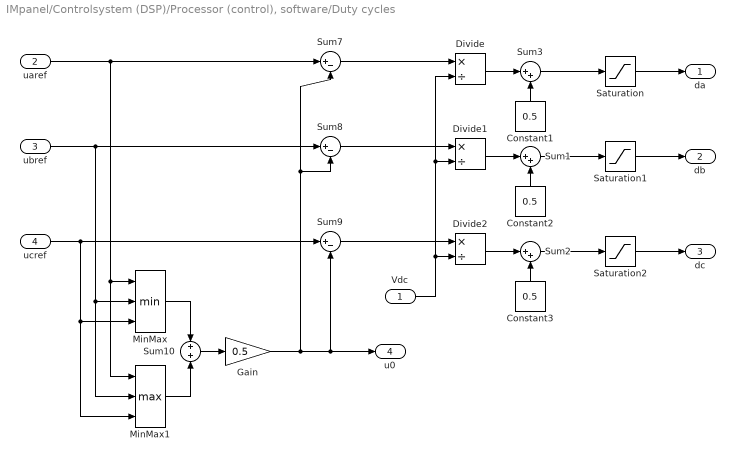
== system IMpanel/Controlsystem (DSP)/Processor (control), software/Duty cycles ==
  Vdc : Inport
  uaref : Inport  Port=2
  ubref : Inport  Port=3
  ucref : Inport  Port=4
  Constant1 : Constant  Value=0.5
  Constant2 : Constant  Value=0.5
  Constant3 : Constant  Value=0.5
  Divide : Product  Inputs=*/
  Divide1 : Product  Inputs=*/
  Divide2 : Product  Inputs=*/
  Gain : Gain  Gain=0.5
  MinMax : MinMax  Inputs=3
  MinMax1 : MinMax  Function=max  Inputs=3
  Saturation : Saturate  UpperLimit=1  LowerLimit=0
  Saturation1 : Saturate  UpperLimit=1  LowerLimit=0
  Saturation2 : Saturate  UpperLimit=1  LowerLimit=0
  Sum1 : Sum  Inputs=|++  SaturateOnIntegerOverflow=on
  Sum10 : Sum  SaturateOnIntegerOverflow=on
  Sum2 : Sum  Inputs=|++  SaturateOnIntegerOverflow=on
  Sum3 : Sum  Inputs=|++  SaturateOnIntegerOverflow=on
  Sum7 : Sum  Inputs=|+-  SaturateOnIntegerOverflow=on
  Sum8 : Sum  Inputs=|+-  SaturateOnIntegerOverflow=on
  Sum9 : Sum  Inputs=|+-  SaturateOnIntegerOverflow=on
  da : Outport  VectorParamsAs1DForOutWhenUnconnected=off
  db : Outport  Port=2  VectorParamsAs1DForOutWhenUnconnected=off
  dc : Outport  Port=3  VectorParamsAs1DForOutWhenUnconnected=off
  u0 : Outport  Port=4  VectorParamsAs1DForOutWhenUnconnected=off
  wires:
  Divide/1 -> Sum3/1
  Constant1/1 -> Sum3/2
  Divide1/1 -> Sum1/1
  Constant2/1 -> Sum1/2
  Divide2/1 -> Sum2/1
  Constant3/1 -> Sum2/2
  Vdc/1 -> Divide/2, Divide1/2, Divide2/2
  Sum3/1 -> Saturation/1
  Sum1/1 -> Saturation1/1
  Sum2/1 -> Saturation2/1
  Sum7/1 -> Divide/1
  Sum9/1 -> Divide2/1
  Sum8/1 -> Divide1/1
  uaref/1 -> Sum7/1, MinMax/1, MinMax1/1
  ubref/1 -> Sum8/1, MinMax1/2, MinMax/2
  ucref/1 -> Sum9/1, MinMax1/3, MinMax/3
  Sum10/1 -> Gain/1
  MinMax/1 -> Sum10/1
  MinMax1/1 -> Sum10/2
  Gain/1 -> Sum8/2, Sum7/2, Sum9/2, u0/1
  Saturation/1 -> da/1
  Saturation1/1 -> db/1
  Saturation2/1 -> dc/1

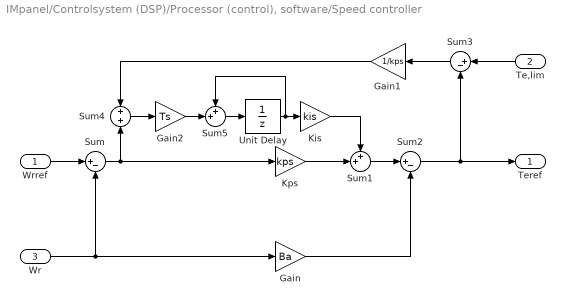
== system IMpanel/Controlsystem (DSP)/Processor (control), software/Speed controller ==
  Wrref : Inport
  Te,lim : Inport  Port=2
  Wr : Inport  Port=3
  Gain : Gain  Gain=Ba
  Gain1 : Gain  Gain=1/kps
  Gain2 : Gain  Gain=Ts
  Kis : Gain  Gain=kis
  Kps : Gain  Gain=kps
  Sum : Sum  Inputs=|+-
  Sum1 : Sum  Inputs=++|
  Sum2 : Sum  Inputs=|+-
  Sum3 : Sum  Inputs=|+-
  Sum4 : Sum
  Sum5 : Sum  Inputs=++|
  Unit Delay : UnitDelay  SampleTime=-1  HasFrameUpgradeWarning=on
  Teref : Outport  VectorParamsAs1DForOutWhenUnconnected=off
  wires:
  Sum4/1 -> Gain2/1
  Gain2/1 -> Sum5/2
  Sum5/1 -> Unit Delay/1
  Kis/1 -> Sum1/1
  Unit Delay/1 -> Sum5/1, Kis/1
  Gain/1 -> Sum2/2
  Kps/1 -> Sum1/2
  Wr/1 -> Gain/1, Sum/2
  Sum3/1 -> Gain1/1
  Sum2/1 -> Teref/1, Sum3/2
  Te,lim/1 -> Sum3/1
  Sum/1 -> Sum4/2, Kps/1
  Sum1/1 -> Sum2/1
  Wrref/1 -> Sum/1
  Gain1/1 -> Sum4/1

== system IMpanel/Controlsystem (DSP)/Processor (control), software/alfa beta to 3 phase ==
  alfa+jbeta : Inport
  Add1 : Sum  Inputs=-+
  Add2 : Sum  Inputs=--
  Complex to Real-Imag : ComplexToRealImag
  Gain1 : Gain  Gain=sqrt(3)/2
  Gain2 : Gain  Gain=1/2
  Xa : Outport  VectorParamsAs1DForOutWhenUnconnected=off
  Xb : Outport  Port=2  VectorParamsAs1DForOutWhenUnconnected=off
  Xc : Outport  Port=3  VectorParamsAs1DForOutWhenUnconnected=off
  wires:
  alfa+jbeta/1 -> Complex to Real-Imag/1
  Complex to Real-Imag/1 -> Xa/1, Gain2/1
  Add2/1 -> Xc/1
  Add1/1 -> Xb/1
  Complex to Real-Imag/2 -> Gain1/1
  Gain1/1 -> Add1/2, Add2/2
  Gain2/1 -> Add1/1, Add2/1

== system IMpanel/Controlsystem (DSP)/Processor (control), software/alfa beta to dq ==
  alfa+jbeta : Inport
  theta : Inport  Port=2
  Gain : Gain  Gain=-j  SaturateOnIntegerOverflow=on  OutDataTypeStr=Inherit: Same as input  ParamDataTypeStr=Inherit: Same as input
  Math Function : Math  SignedPower=on  SaturateOnIntegerOverflow=on
  Product : Product  SaturateOnIntegerOverflow=on  OutDataTypeStr=Inherit: Same as first input
  d+jq : Outport  VectorParamsAs1DForOutWhenUnconnected=off
  wires:
  theta/1 -> Gain/1
  Gain/1 -> Math Function/1
  Math Function/1 -> Product/2
  alfa+jbeta/1 -> Product/1
  Product/1 -> d+jq/1

== system IMpanel/Controlsystem (DSP)/Processor (control), software/dq to alfa beta ==
  d+jq : Inport
  theta : Inport  Port=2
  Gain : Gain  Gain=j  SaturateOnIntegerOverflow=on  OutDataTypeStr=Inherit: Same as input  ParamDataTypeStr=Inherit: Same as input
  Math Function : Math  SignedPower=on  SaturateOnIntegerOverflow=on
  Product : Product  SaturateOnIntegerOverflow=on  OutDataTypeStr=Inherit: Same as first input
  alfa+jbeta : Outport  VectorParamsAs1DForOutWhenUnconnected=off
  wires:
  theta/1 -> Gain/1
  Gain/1 -> Math Function/1
  Math Function/1 -> Product/2
  d+jq/1 -> Product/1
  Product/1 -> alfa+jbeta/1
